simulink model "control2"  (R2018a)
settings: Solver=VariableStepAuto  StartTime=0.0  StopTime=16  RelTol=1e-3
values from neighbouring files (symbols this model uses):
  CT1 = [C1 0]    [values.m]
  CT2 = [C2 0]    [values.m]
  dnorm = 0.09/(0.3-0.09) * dnorm    (= 0.428571428571)    [values.m]
  g = 9.81    [values.m]
  gammaT1 = [ ... (first row only)    [values.m]
  gammaT2 = [ ... (first row only)    [values.m]
  GT1 = GTt1'    [values.m]
  GT2 = GTt2'    [values.m]
  K1 = acker(phi1, gamma1, [zDominant1, zDominant2, zcinf, zcinf])    [values.m]
  K2 = acker(phi2, gamma2, [zDominant1, zDominant2])    [values.m]
  m = 5    [values.m]
  M = 1.8    [values.m]
  Nu1 = N1(end)    [values.m]
  Nu2 = N2(end)    [values.m]
  Nx2 = N2(1:2)    [values.m]
  P = 0.04    [values.m]
  phiT1 = [ ... (first row only)    [values.m]
  phiT2 = [ ... (first row only)    [values.m]
  T = 1/(5*abs(soinf))    [values.m]
  Tdstart = 4    [values.m]
  y0 = 0.9    [values.m]
undefined symbols (not defined in the file or in its folder): C1, C2, D1, D2, gamma1, gamma2, Nx1, phi1, phi2
settings Model: Creator=cloud  LastModifiedBy=cloud

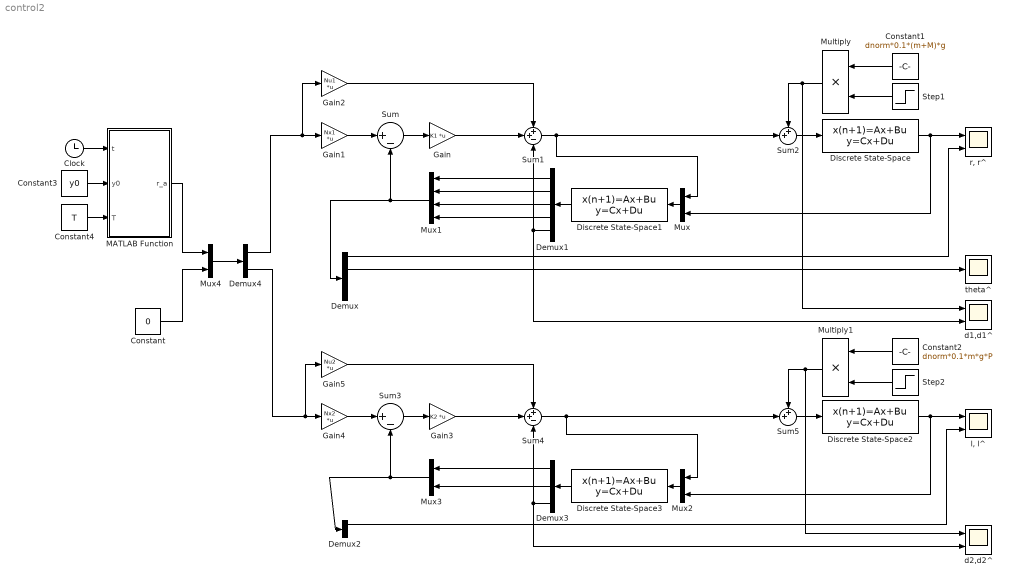
== system control2 ==
  Clock : Clock
  Constant : Constant  Value=0
  Constant1 : Constant  Value=dnorm*0.1*(m+M)*g
  Constant2 : Constant  Value=dnorm*0.1*m*g*P
  Constant3 : Constant  Value=y0
  Constant4 : Constant  Value=T
  Demux : Demux
  Demux1 : Demux  Outputs=5
  Demux2 : Demux  Outputs=2
  Demux3 : Demux  Outputs=3
  Demux4 : Demux  Outputs=2
  Discrete State-Space : DiscreteStateSpace  A=phi1  B=gamma1  C=C1  D=D1  InitialCondition=[0; 0; 0; 0]  SampleTime=T
  Discrete State-Space1 : DiscreteStateSpace  A=phiT1-GT1*CT1*phiT1  B=[(gammaT1-GT1*CT1*gammaT1) GT1]  C=eye(5)  D=zeros(5,2)  SampleTime=T
  Discrete State-Space2 : DiscreteStateSpace  A=phi2  B=gamma2  C=C2  D=D2  InitialCondition=[0; 0]  SampleTime=T
  Discrete State-Space3 : DiscreteStateSpace  A=phiT2-GT2*CT2*phiT2  B=[(gammaT2-GT2*CT2*gammaT2) GT2]  C=eye(3)  D=zeros(3,2)  SampleTime=T
  Gain : Gain  Gain=K1  Multiplication=Matrix(K*u)
  Gain1 : Gain  Gain=Nx1  Multiplication=Matrix(K*u)
  Gain2 : Gain  Gain=Nu1  Multiplication=Matrix(K*u)
  Gain3 : Gain  Gain=K2  Multiplication=Matrix(K*u)
  Gain4 : Gain  Gain=Nx2  Multiplication=Matrix(K*u)
  Gain5 : Gain  Gain=Nu2  Multiplication=Matrix(K*u)
  MATLAB Function : MATLAB Function  TreatAsAtomicUnit=on
  Multiply : Product
  Multiply1 : Product
  Mux{,2..4} (4 alike) : Mux  Inputs=2
  Mux1 : Mux
  Step1 : Step  Time=Tdstart  SampleTime=T
  Step2 : Step  Time=Tdstart  SampleTime=T
  Sum : Sum  Inputs=|+-
  Sum1 : Sum  Inputs=++-
  Sum2 : Sum  Inputs=++|
  Sum3 : Sum  Inputs=|+-
  Sum4 : Sum  Inputs=++-
  Sum5 : Sum  Inputs=++|
  d1,d1^ : Scope  NumInputPorts=2
  d2,d2^ : Scope  NumInputPorts=2
  "l, l^" : Scope  NumInputPorts=2
  "r, r^" : Scope  NumInputPorts=2
  theta^ : Scope
  wires:
  Mux/1 -> Discrete State-Space1/1
  Discrete State-Space/1 -> Mux/2, "r, r^"/1
  Demux/1 -> "r, r^"/2
  Gain1/1 -> Sum/1
  Sum/1 -> Gain/1
  Gain/1 -> Sum1/2
  Gain2/1 -> Sum1/1
  Discrete State-Space1/1 -> Demux1/1
  Demux1/5 -> d1,d1^/2, Sum1/3
  Sum2/1 -> Discrete State-Space/1
  Multiply/1 -> d1,d1^/1, Sum2/1
  Demux1/1 -> Mux1/1
  Demux1/2 -> Mux1/2
  Demux1/3 -> Mux1/3
  Demux1/4 -> Mux1/4
  Mux1/1 -> Sum/2, Demux/1
  Demux/2 -> theta^/1
  Multiply1/1 -> Sum5/1, d2,d2^/1
  Mux3/1 -> Demux2/1, Sum3/2
  Demux3/3 -> d2,d2^/2, Sum4/3
  Sum5/1 -> Discrete State-Space2/1
  Discrete State-Space3/1 -> Demux3/1
  Demux3/1 -> Mux3/1
  Gain3/1 -> Sum4/2
  Sum3/1 -> Gain3/1
  Demux3/2 -> Mux3/2
  Gain4/1 -> Sum3/1
  Discrete State-Space2/1 -> Mux2/2, "l, l^"/1
  Demux4/1 -> Gain2/1, Gain1/1
  Demux2/1 -> "l, l^"/2
  Mux2/1 -> Discrete State-Space3/1
  Gain5/1 -> Sum4/1
  MATLAB Function/1(r_a) -> Mux4/1
  Mux4/1 -> Demux4/1
  Demux4/2 -> Gain5/1, Gain4/1
  Constant/1 -> Mux4/2
  Sum1/1 -> Mux/1, Sum2/2
  Sum4/1 -> Mux2/1, Sum5/2
  Clock/1 -> MATLAB Function/1(t)
  Step1/1 -> Multiply/2
  Constant1/1 -> Multiply/1
  Step2/1 -> Multiply1/2
  Constant2/1 -> Multiply1/1
  Constant3/1 -> MATLAB Function/2(y0)
  Constant4/1 -> MATLAB Function/3(T)

== matlab function control2/MATLAB Function ==
  data: t input; r_a output; y0 input; T input
function r_a = fcn(t, y0, T)

r_a = 0.1*y0*(1-exp(-t/T));
